simulink model "first_order_low_pass_filtering"  (R2023b)
settings: Solver=VariableStepAuto  StartTime=0.0  StopTime=10.0  RelTol=1e-3
libraries: dspfdesign x2
settings Model: Creator=JHHK-SJM  LastModifiedBy=JUEMING_SHI

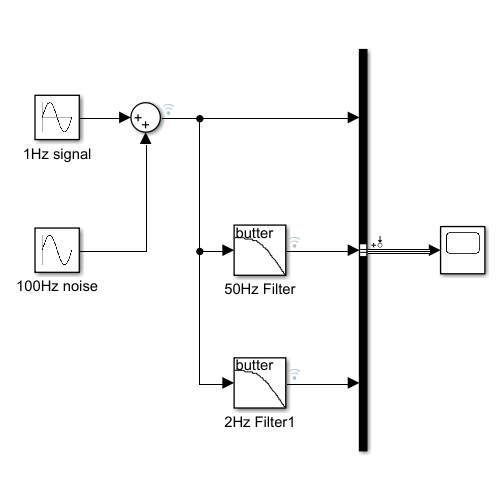
[thumbnail: Simulink's stored preview of the top-level diagram]
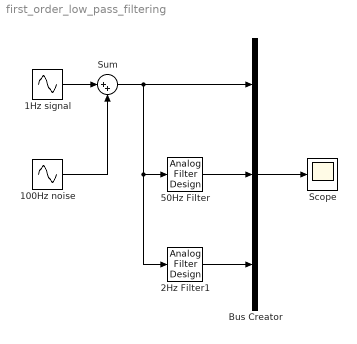
== system first_order_low_pass_filtering ==
  100Hz noise : Sin  Amplitude=0.3  Frequency=200*pi  SampleTime=0
  1Hz signal : Sin  Frequency=2*pi  SampleTime=0
  2Hz Filter1 : dspfdesign/Analog Filter Design  method=Butterworth  filttype=Lowpass  N=1  Wlo=4*pi  Whi=80  Rp=2  Rs=40
  50Hz Filter : dspfdesign/Analog Filter Design  method=Butterworth  filttype=Lowpass  N=1  Wlo=100*pi  Whi=80  Rp=2  Rs=40
  Bus Creator : BusCreator  Inputs=3
  Scope : Scope
  Sum : Sum  Inputs=|++
  wires:
  1Hz signal/1 -> Sum/1
  100Hz noise/1 -> Sum/2
  Sum/1 -> 2Hz Filter1/1, 50Hz Filter/1, Bus Creator/1
  50Hz Filter/1 -> Bus Creator/2
  Bus Creator/1 -> Scope/1
  2Hz Filter1/1 -> Bus Creator/3
